simulink model "adc16_dbf_4fft"  (R2013a)
settings: Solver=ode45  StartTime=0.0  StopTime=2050  RelTol=1e-3
undefined symbols (not defined in the file): pfb_coeff_gen_calc
libraries: xbsIndex_r4 x1713, casper_library_misc x294, casper_library_delays x48, casper_library_pfbs x16, simulink x16, xps_library x1
(part 1 of 21)
settings Model: Creator=root  LastModifiedBy=root

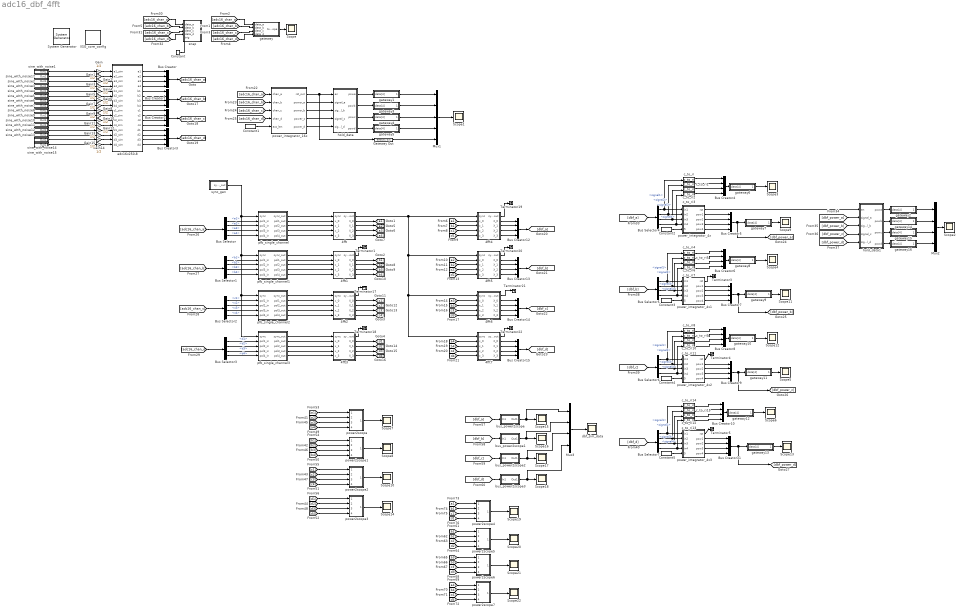
== system adc16_dbf_4fft ==
  " System Generator" : xbsIndex_r4/ System Generator  Tag=genX  xilinxfamily=Kintex7  part=xc7k325t  speed=-3  package=fbg676  synthesis_tool=XST  clock_wrapper=Clock Enables  directory=./netlist  proj_type=Project Navigator  Synth_file=XST Defaults  Impl_file=ISE Defaults  testbench=off  simulink_period=1  sysclk_period=10  dcm_input_clock_period=10  incr_netlist=off  trim_vbits=Everywhere in SubSystem  dbl_ovrd=According to Block Masks  core_generation=According to Block Masks  run_coregen=off  deprecated_control=off  eval_field=0  block_type=sysgen
  4fft : Subsystem
  4fft1 : Subsystem
  4fft2 : Subsystem
  4fft3 : Subsystem
  4fft4 : Subsystem
  4fft5 : Subsystem
  4fft6 : Subsystem
  4fft7 : Subsystem
  Bus Creator{,1..15} (16 alike) : BusCreator
  Bus Selector : BusSelector  OutputSignals=a1,a2,a3,a4
  Bus Selector1 : BusSelector  OutputSignals=b1,b2,b3,b4
  Bus Selector2 : BusSelector  OutputSignals=c1,c2,c3,c4
  Bus Selector3 : BusSelector  OutputSignals=d1,d2,d3,d4
  Bus Selector{4..7} (4 alike) : BusSelector  OutputSignals=signal1,signal2,signal3,signal4
  Constant : xbsIndex_r4/Constant  const=1  gui_display_data_type=Boolean  arith_type=Boolean  n_bits=16  bin_pt=14  preci_type=Single  exp_width=8  frac_width=24  explicit_period=off  period=1  equ=P=C  opselect=C  inp2=PCIN>>17  opr=+  inp1=P  carry=CIN  dbl_ovrd=off  block_type=constant
  Constant1 : xbsIndex_r4/Constant  const=255  gui_display_data_type=Fixed-point  arith_type=Unsigned  n_bits=10  bin_pt=0  preci_type=Single  exp_width=8  frac_width=24  explicit_period=off  period=1  equ=P=C  opselect=C  inp2=PCIN>>17  opr=+  inp1=P  carry=CIN  dbl_ovrd=off  block_type=constant
  Constant{2..5} (4 alike) : xbsIndex_r4/Constant  const=511  gui_display_data_type=Fixed-point  arith_type=Unsigned  n_bits=10  bin_pt=0  preci_type=Single  exp_width=8  frac_width=24  explicit_period=off  period=1  equ=P=C  opselect=C  inp2=PCIN>>17  opr=+  inp1=P  carry=CIN  dbl_ovrd=off  block_type=constant
  Gain{,1..15} (16 alike) : Gain  Gain=1/2
  Gateway Out : xbsIndex_r4/Gateway Out  inherit_from_input=off  hdl_port=on  timing_constraint=None  locs_specified=off  LOCs={}  UseAsDAC=off  DACChannel='1'  block_type=gatewayout
  Mux1 : Mux  Inputs=5
  Mux2 : Mux
  Mux3 : Mux
  Scope{,1..22} (23 alike) : Scope
      Scope10 settings: SaveName=ScopeData10
      Scope11 settings: SaveName=ScopeData4
      Scope12 settings: SaveName=ScopeData6
      Scope13 settings: SaveName=ScopeData7
      Scope14 settings: SaveName=ScopeData14
      Scope15 settings: SaveName=ScopeData15
      Scope16 settings: SaveName=ScopeData16
      Scope17 settings: SaveName=ScopeData17
      Scope18 settings: SaveName=ScopeData18
      Scope19 settings: SaveName=ScopeData19
      Scope2 settings: SaveName=ScopeData2
      Scope20 settings: SaveName=ScopeData20
      Scope21 settings: SaveName=ScopeData21
      Scope22 settings: SaveName=ScopeData22
      Scope3 settings: SaveName=ScopeData3
      Scope4 settings: SaveName=ScopeData11
      Scope5 settings: SaveName=ScopeData12
      Scope6 settings: SaveName=ScopeData13
      Scope7 settings: SaveName=ScopeData5
      Scope8 settings: SaveName=ScopeData8
      Scope9 settings: SaveName=ScopeData9
  Terminator{1,3..5,17..22} (10 alike) : Terminator
  XSG_core_config : xps_library/XSG_core_config  Tag=xps:xsg  hw_sys=ROACH2:sx475t  clk_src=adc0_clk  ROACH_clk_src=sys_clk  ROACH2_clk_src=adc0_clk  MKDIG_clk_src=sys_clk  clk_rate=240  sample_period=1  synthesis_tool=XST
  adc16x250-8 : Subsystem  Tag=xps:adc16  AncestorBlock=xps_library/ADCs/adc16x250-8  mask(ADC16){board_count=1, roach2_rev=2, zdok_rev=2}
      mask prompts: board_count "Number of ADC16 Boards"; roach2_rev "ROACH2 Revision"; zdok_rev "ZDOK Pinout Revision"
      mask help: 16-input ADC. When using one ADC16 board, it must be in ZDOK0.
      mask init:
      | % Only board_count is needed by init function
      | adc16_init(gcb, ...
      |     'board_count', board_count);
      settings: AttributesFormatString=r2 rev%<roach2_rev>\nzdok rev%<zdok_rev>
      mask Help:
      | This is the CASPER "yellow block" for the CASPER ADC16 board.  Each ADC
      | board has four ADC chips.  Each ADC chip accepts four inputs.  The four
      | 8-bit outputs from each ADC chip are concatenated into a 32-bit signal.
      mask TypeOptions board_count: 1 | 2
      mask TypeOptions roach2_rev: 1 | 2
      mask TypeOptions zdok_rev: 1 | 2
  bus_power2scope : Subsystem
  bus_power2scope1 : Subsystem
  bus_power2scope2 : Subsystem
  bus_power2scope3 : Subsystem
  c_to_ri{,1..15} (16 alike) : casper_library_misc/c_to_ri  n_bits=18  bin_pt=17
  dbf_sim_data : Scope
      settings: SaveName=dbf_sim_data
  gateway : Subsystem
  gateway1 : Subsystem
  gateway10 : Subsystem
  gateway11 : Subsystem
  gateway12 : Subsystem
  gateway13 : Subsystem
  gateway14 : Subsystem
  gateway15 : Subsystem
  gateway16 : Subsystem
  gateway2 : Subsystem
  gateway3 : Subsystem
  gateway4 : Subsystem
  gateway5 : Subsystem
  gateway6 : Subsystem
  gateway7 : Subsystem
  gateway8 : Subsystem
  gateway9 : Subsystem
  hold_data : Subsystem
  hold_data1 : Subsystem
  pfb_single_channel : Subsystem
  pfb_single_channel1 : Subsystem
  pfb_single_channel2 : Subsystem
  pfb_single_channel3 : Subsystem
  power2scope : Subsystem
  power2scope1 : Subsystem
  power2scope2 : Subsystem
  power2scope3 : Subsystem
  power2scope4 : Subsystem
  power2scope5 : Subsystem
  power2scope6 : Subsystem
  power2scope7 : Subsystem
  power_integrator_16x : Subsystem
  power_integrator_4x : Subsystem
  power_integrator_4x1 : Subsystem
  power_integrator_4x2 : Subsystem
  power_integrator_4x3 : Subsystem
  sine_with_noise1 : Subsystem
  sine_with_noise10 : Subsystem
  sine_with_noise11 : Subsystem
  sine_with_noise12 : Subsystem
  sine_with_noise13 : Subsystem
  sine_with_noise14 : Subsystem
  sine_with_noise15 : Subsystem
  sine_with_noise17 : Subsystem
  sine_with_noise2 : Subsystem
  sine_with_noise3 : Subsystem
  sine_with_noise4 : Subsystem
  sine_with_noise5 : Subsystem
  sine_with_noise6 : Subsystem
  sine_with_noise7 : Subsystem
  sine_with_noise8 : Subsystem
  sine_with_noise9 : Subsystem
  snap : Subsystem
  sync_gen : Subsystem  AncestorBlock=casper_library_misc/sync_gen  mask(sync_gen){sim_acc_len=4, fft_size=4, fft_simult_inputs=1, pfb_fir_taps=1, reorder_vec=[2 2 2], scale=32}
      mask prompts: sim_acc_len "Simulation Accumulation Length"; fft_size "FFT Size"; fft_simult_inputs "Simultaneous Inputs (FFT)"; pfb_fir_taps "Taps in pfb_fir (use 1 if no pfb_fir)"; reorder_vec "Reorder Orders (e.g. [2 2 2])"
      mask help:
      | This block computes the sync period based on system parameters as
      | described in Casper memo.  Detailed descritions of the block's
      | variables can be found in the 'Block Documentation' section of
      | the CASPER wiki.
      mask init:
      | sync_gen_init(gcb, ...
      |     'sim_acc_len', sim_acc_len, ...
      |     'fft_size', fft_size, ...
      |     'fft_simult_inputs', fft_simult_inputs,...
      |     'pfb_fir_taps', pfb_fir_taps, ...
      |     'reorder_vec', reorder_vec, ...
      |     'scale', scale);
      settings: AttributesFormatString=sim_sync_period=1024
      mask Help:
      | SyncPeriod=LCM(reorder_vec)*(acc_num)*(pfb_fir_len)*(fft_size/fft_simult_inputs)
      | 
      | See CASPER sync pulse memo for more details.
  wires:
  adc16x250-8/3(a3) -> Bus Creator/3
  adc16x250-8/2(a2) -> Bus Creator/2
  adc16x250-8/4(a4) -> Bus Creator/4
  Constant/1 -> snap/5(trig)
  gateway/1(to_scope) -> Scope/1
  sine_with_noise1/1(Out1) -> Gain/1
  Gain/1 -> adc16x250-8/1(a1_sim)
  Gain1/1 -> adc16x250-8/2(a2_sim)
  Gain2/1 -> adc16x250-8/3(a3_sim)
  Gain3/1 -> adc16x250-8/4(a4_sim)
  Gain4/1 -> adc16x250-8/5(b1_sim)
  Gain5/1 -> adc16x250-8/6(b2_sim)
  Gain6/1 -> adc16x250-8/7(b3_sim)
  Gain7/1 -> adc16x250-8/8(b4_sim)
  Gain10/1 -> adc16x250-8/11(c3_sim)
  Gain8/1 -> adc16x250-8/9(c1_sim)
  Gain12/1 -> adc16x250-8/13(d1_sim)
  Gain15/1 -> adc16x250-8/16(d4_sim)
  Gain11/1 -> adc16x250-8/12(c4_sim)
  Gain14/1 -> adc16x250-8/15(d3_sim)
  Gain9/1 -> adc16x250-8/10(c2_sim)
  Gain13/1 -> adc16x250-8/14(d2_sim)
  adc16x250-8/1(a1) -> Bus Creator/1
  Bus Creator/1 -> [adc16_chan_a]
  power_integrator_16x/2(power_a) -> hold_data/2(signal_a)
  hold_data/1(powa) -> gateway1/1(data[4])
  power_integrator_16x/1(rst_out) -> Gateway Out/1, hold_data/1(en)
  Mux1/1 -> Scope1/1
  Gateway Out/1 -> Mux1/5
  [adc16_chan_a] -> Bus Selector/1
  [adc16_chan_a] -> gateway/1(data_a)
  sync_gen/1(sync_out) -> pfb_single_channel3/1(sync), pfb_single_channel2/1(sync), pfb_single_channel1/1(sync), pfb_single_channel/1(sync)
  Bus Selector/4 -> pfb_single_channel/5(pol4_in)  "<a4>"
  Bus Selector/2 -> pfb_single_channel/3(pol2_in)  "<a2>"
  Bus Selector/1 -> pfb_single_channel/2(pol1_in)  "<a1>"
  Bus Selector/3 -> pfb_single_channel/4(pol3_in)  "<a3>"
  sine_with_noise17/1(Out1) -> Gain1/1
  sine_with_noise2/1(Out1) -> Gain2/1
  sine_with_noise3/1(Out1) -> Gain3/1
  sine_with_noise4/1(Out1) -> Gain4/1
  sine_with_noise5/1(Out1) -> Gain5/1
  sine_with_noise6/1(Out1) -> Gain6/1
  sine_with_noise7/1(Out1) -> Gain7/1
  sine_with_noise8/1(Out1) -> Gain8/1
  sine_with_noise9/1(Out1) -> Gain9/1
  sine_with_noise10/1(Out1) -> Gain10/1
  sine_with_noise11/1(Out1) -> Gain11/1
  sine_with_noise12/1(Out1) -> Gain12/1
  sine_with_noise13/1(Out1) -> Gain13/1
  sine_with_noise14/1(Out1) -> Gain14/1
  sine_with_noise15/1(Out1) -> Gain15/1
  pfb_single_channel/1(sync_out) -> 4fft/1(sync)
  4fft/1(sync_out) -> 4fft4/1(sync), 4fft5/1(sync), 4fft6/1(sync), 4fft7/1(sync)
  [adc16_chan_b] -> Bus Selector1/1
  pfb_single_channel1/2(pol1_out) -> 4fft1/2(x_0)
  pfb_single_channel1/4(pol3_out) -> 4fft1/4(x_2)
  pfb_single_channel1/3(pol2_out) -> 4fft1/3(x_1)
  pfb_single_channel1/5(pol4_out) -> 4fft1/5(x_3)
  Bus Selector1/4 -> pfb_single_channel1/5(pol4_in)  "<b4>"
  Bus Selector1/2 -> pfb_single_channel1/3(pol2_in)  "<b2>"
  Bus Selector1/1 -> pfb_single_channel1/2(pol1_in)  "<b1>"
  Bus Selector1/3 -> pfb_single_channel1/4(pol3_in)  "<b3>"
  pfb_single_channel1/1(sync_out) -> 4fft1/1(sync)
  4fft1/1(sync_out) -> Terminator1/1
  [adc16_chan_c] -> Bus Selector2/1
  pfb_single_channel2/2(pol1_out) -> 4fft2/2(x_0)
  pfb_single_channel2/4(pol3_out) -> 4fft2/4(x_2)
  pfb_single_channel2/3(pol2_out) -> 4fft2/3(x_1)
  pfb_single_channel2/5(pol4_out) -> 4fft2/5(x_3)
  Bus Selector2/4 -> pfb_single_channel2/5(pol4_in)  "<c4>"
  Bus Selector2/2 -> pfb_single_channel2/3(pol2_in)  "<c2>"
  Bus Selector2/1 -> pfb_single_channel2/2(pol1_in)  "<c1>"
  Bus Selector2/3 -> pfb_single_channel2/4(pol3_in)  "<c3>"
  pfb_single_channel2/1(sync_out) -> 4fft2/1(sync)
  4fft2/1(sync_out) -> Terminator17/1
  [adc16_chan_d] -> Bus Selector3/1
  pfb_single_channel3/2(pol1_out) -> 4fft3/2(x_0)
  pfb_single_channel3/4(pol3_out) -> 4fft3/4(x_2)
  pfb_single_channel3/3(pol2_out) -> 4fft3/3(x_1)
  pfb_single_channel3/5(pol4_out) -> 4fft3/5(x_3)
  Bus Selector3/4 -> pfb_single_channel3/5(pol4_in)  "<d4>"
  Bus Selector3/2 -> pfb_single_channel3/3(pol2_in)  "<d2>"
  Bus Selector3/1 -> pfb_single_channel3/2(pol1_in)  "<d1>"
  Bus Selector3/3 -> pfb_single_channel3/4(pol3_in)  "<d3>"
  pfb_single_channel3/1(sync_out) -> 4fft3/1(sync)
  4fft3/1(sync_out) -> Terminator18/1
  4fft/5(X_3) -> [a4]
  4fft/2(X_0) -> [a1]
  4fft/4(X_2) -> [a3]
  4fft/3(X_1) -> [a2]
  4fft2/3(X_1) -> [c2]
  4fft2/2(X_0) -> [c1]
  4fft2/4(X_2) -> [c3]
  4fft2/5(X_3) -> [c4]
  4fft3/2(X_0) -> [d1]
  4fft3/3(X_1) -> [d2]
  4fft3/4(X_2) -> [d3]
  4fft3/5(X_3) -> [d4]
  4fft1/2(X_0) -> [b1]
  4fft1/3(X_1) -> [b2]
  4fft1/4(X_2) -> [b3]
  4fft1/5(X_3) -> [b4]
  [a1] -> 4fft4/2(x_0)
  [b1] -> 4fft4/3(x_1)
  [c1] -> 4fft4/4(x_2)
  [d1] -> 4fft4/5(x_3)
  4fft4/1(sync_out) -> Terminator19/1
  [a2] -> 4fft5/2(x_0)
  [b2] -> 4fft5/3(x_1)
  [c2] -> 4fft5/4(x_2)
  [d2] -> 4fft5/5(x_3)
  [a3] -> 4fft6/2(x_0)
  [b3] -> 4fft6/3(x_1)
  [c3] -> 4fft6/4(x_2)
  [d3] -> 4fft6/5(x_3)
  [a4] -> 4fft7/2(x_0)
  [b4] -> 4fft7/3(x_1)
  [c4] -> 4fft7/4(x_2)
  [d4] -> 4fft7/5(x_3)
  4fft5/1(sync_out) -> Terminator20/1
  4fft6/1(sync_out) -> Terminator21/1
  4fft7/1(sync_out) -> Terminator22/1
  Constant1/1 -> power_integrator_16x/5(acc_len)
  adc16x250-8/8(b4) -> Bus Creator1/4
  adc16x250-8/6(b2) -> Bus Creator1/2
  adc16x250-8/7(b3) -> Bus Creator1/3
  adc16x250-8/5(b1) -> Bus Creator1/1
  adc16x250-8/12(c4) -> Bus Creator2/4
  adc16x250-8/11(c3) -> Bus Creator2/3
  adc16x250-8/10(c2) -> Bus Creator2/2
  adc16x250-8/9(c1) -> Bus Creator2/1
  adc16x250-8/15(d3) -> Bus Creator3/3
  adc16x250-8/16(d4) -> Bus Creator3/4
  adc16x250-8/14(d2) -> Bus Creator3/2
  adc16x250-8/13(d1) -> Bus Creator3/1
  Bus Creator1/1 -> [adc16_chan_b]
  Bus Creator2/1 -> [adc16_chan_c]
  Bus Creator3/1 -> [adc16_chan_d]
  [adc16_chan_a] -> power_integrator_16x/1(chan_a)
  [adc16_chan_b] -> power_integrator_16x/2(chan_b)
  [adc16_chan_c] -> power_integrator_16x/3(chan_c)
  [adc16_chan_d] -> power_integrator_16x/4(chan_d)
  power_integrator_16x/3(power_b) -> hold_data/3(signal_b)
  power_integrator_16x/4(power_c) -> hold_data/4(signal_c)
  power_integrator_16x/5(power_d) -> hold_data/5(signal_d)
  hold_data/2(powb) -> gateway3/1(data[4])
  hold_data/3(powc) -> gateway4/1(data[4])
  hold_data/4(powd) -> gateway5/1(data[4])
  gateway1/1(to_scope) -> Mux1/1
  gateway3/1(to_scope) -> Mux1/2
  gateway4/1(to_scope) -> Mux1/3
  gateway5/1(to_scope) -> Mux1/4
  [adc16_chan_b] -> gateway/2(data_b)
  [adc16_chan_c] -> gateway/3(data_c)
  [adc16_chan_d] -> gateway/4(data_d)
  [adc16_chan_c] -> snap/3(data_c)
  [adc16_chan_b] -> snap/2(data_b)
  [adc16_chan_d] -> snap/4(data_d)
  [adc16_chan_a] -> snap/1(data_a)
  pfb_single_channel/2(pol1_out) -> 4fft/2(x_0)
  pfb_single_channel/3(pol2_out) -> 4fft/3(x_1)
  pfb_single_channel/4(pol3_out) -> 4fft/4(x_2)
  pfb_single_channel/5(pol4_out) -> 4fft/5(x_3)
  Constant2/1 -> power_integrator_4x/5(acc_len)
  power_integrator_4x/1(rst) -> hold_data1/1(en)
  4fft4/3(X_1) -> Bus Creator12/2
  4fft4/4(X_2) -> Bus Creator12/3
  4fft4/2(X_0) -> Bus Creator12/1
  4fft4/5(X_3) -> Bus Creator12/4
  4fft5/5(X_3) -> Bus Creator13/4
  4fft5/4(X_2) -> Bus Creator13/3
  4fft5/2(X_0) -> Bus Creator13/1
  4fft5/3(X_1) -> Bus Creator13/2
  4fft6/2(X_0) -> Bus Creator14/1
  4fft6/3(X_1) -> Bus Creator14/2
  4fft6/4(X_2) -> Bus Creator14/3
  4fft6/5(X_3) -> Bus Creator14/4
  4fft7/5(X_3) -> Bus Creator15/4
  4fft7/2(X_0) -> Bus Creator15/1
  4fft7/3(X_1) -> Bus Creator15/2
  4fft7/4(X_2) -> Bus Creator15/3
  Bus Creator12/1 -> [dbf_a]
  Bus Creator13/1 -> [dbf_b]
  Bus Creator15/1 -> [dbf_d]
  [dbf_a] -> Bus Selector4/1
  [dbf_b] -> Bus Selector5/1
  [dbf_c] -> Bus Selector6/1
  [dbf_d] -> Bus Selector7/1
  Bus Selector4/1 -> c_to_ri/1, power_integrator_4x/1(in1)  "<signal1>"
  Bus Selector4/2 -> c_to_ri1/1, power_integrator_4x/2(in2)  "<signal2>"
  Bus Selector4/3 -> c_to_ri2/1, power_integrator_4x/3(in3)  "<signal3>"
  Bus Selector4/4 -> c_to_ri3/1, power_integrator_4x/4(in4)  "<signal4>"
  Constant3/1 -> power_integrator_4x1/5(acc_len)
  power_integrator_4x1/1(rst) -> Terminator3/1
  Bus Selector5/3 -> c_to_ri6/1, power_integrator_4x1/3(in3)  "<signal3>"
  Bus Selector5/2 -> c_to_ri5/1, power_integrator_4x1/2(in2)  "<signal2>"
  Bus Selector5/4 -> c_to_ri7/1, power_integrator_4x1/4(in4)  "<signal4>"
  Bus Selector5/1 -> power_integrator_4x1/1(in1), c_to_ri4/1  "<signal1>"
  Constant4/1 -> power_integrator_4x2/5(acc_len)
  power_integrator_4x2/1(rst) -> Terminator4/1
  Bus Selector6/3 -> c_to_ri10/1, power_integrator_4x2/3(in3)  "<signal3>"
  Bus Selector6/2 -> c_to_ri9/1, power_integrator_4x2/2(in2)  "<signal2>"
  Bus Selector6/4 -> c_to_ri11/1, power_integrator_4x2/4(in4)  "<signal4>"
  Bus Selector6/1 -> c_to_ri8/1, power_integrator_4x2/1(in1)  "<signal1>"
  Constant5/1 -> power_integrator_4x3/5(acc_len)
  power_integrator_4x3/1(rst) -> Terminator5/1
  Bus Selector7/3 -> c_to_ri12/1, power_integrator_4x3/3(in3)  "<signal3>"
  Bus Selector7/2 -> c_to_ri15/1, power_integrator_4x3/2(in2)  "<signal2>"
  Bus Selector7/4 -> c_to_ri13/1, power_integrator_4x3/4(in4)  "<signal4>"
  Bus Selector7/1 -> c_to_ri14/1, power_integrator_4x3/1(in1)  "<signal1>"
  power_integrator_4x/5(pow4) -> Bus Creator5/4
  power_integrator_4x/3(pow2) -> Bus Creator5/2
  power_integrator_4x/2(pow1) -> Bus Creator5/1
  power_integrator_4x/4(pow3) -> Bus Creator5/3
  Bus Creator4/1 -> gateway6/1(data[4])
  gateway6/1(to_scope) -> Scope3/1
  gateway7/1(to_scope) -> Scope9/1
  Bus Creator5/1 -> [dbf_power_a], gateway7/1(data[4])
  power_integrator_4x1/5(pow4) -> Bus Creator7/4
  power_integrator_4x1/3(pow2) -> Bus Creator7/2
  power_integrator_4x1/2(pow1) -> Bus Creator7/1
  power_integrator_4x1/4(pow3) -> Bus Creator7/3
  Bus Creator6/1 -> gateway8/1(data[4])
  gateway8/1(to_scope) -> Scope4/1
  gateway9/1(to_scope) -> Scope11/1
  Bus Creator7/1 -> [dbf_power_b], gateway9/1(data[4])
  power_integrator_4x2/5(pow4) -> Bus Creator9/4
  power_integrator_4x2/3(pow2) -> Bus Creator9/2
  power_integrator_4x2/2(pow1) -> Bus Creator9/1
  power_integrator_4x2/4(pow3) -> Bus Creator9/3
  Bus Creator8/1 -> gateway10/1(data[4])
  gateway10/1(to_scope) -> Scope12/1
  gateway11/1(to_scope) -> Scope5/1
  power_integrator_4x3/5(pow4) -> Bus Creator11/4
  power_integrator_4x3/3(pow2) -> Bus Creator11/2
  power_integrator_4x3/2(pow1) -> Bus Creator11/1
  power_integrator_4x3/4(pow3) -> Bus Creator11/3
  Bus Creator10/1 -> gateway12/1(data[4])
  gateway12/1(to_scope) -> Scope6/1
  gateway13/1(to_scope) -> Scope13/1
  Bus Creator14/1 -> [dbf_c]
  c_to_ri/1 -> Bus Creator4/1
  c_to_ri4/2 -> Bus Creator6/1
  c_to_ri5/2 -> Bus Creator6/2
  c_to_ri6/2 -> Bus Creator6/3
  c_to_ri7/2 -> Bus Creator6/4
  c_to_ri11/2 -> Bus Creator8/4
  c_to_ri10/2 -> Bus Creator8/3
  c_to_ri9/2 -> Bus Creator8/2
  c_to_ri8/2 -> Bus Creator8/1
  c_to_ri13/2 -> Bus Creator10/4
  c_to_ri12/2 -> Bus Creator10/3
  c_to_ri15/2 -> Bus Creator10/2
  c_to_ri14/2 -> Bus Creator10/1
  Bus Creator9/1 -> [dbf_power_c], gateway11/1(data[4])
  Bus Creator11/1 -> [dbf_power_d], gateway13/1(data[4])
  [dbf_power_a] -> hold_data1/2(signal_a)
  [dbf_power_b] -> hold_data1/3(signal_b)
  [dbf_power_c] -> hold_data1/4(signal_c)
  [dbf_power_d] -> hold_data1/5(signal_d)
  gateway2/1(to_scope) -> Mux2/1
  gateway14/1(to_scope) -> Mux2/2
  gateway15/1(to_scope) -> Mux2/3
  gateway16/1(to_scope) -> Mux2/4
  hold_data1/1(powa) -> gateway2/1(data[4])
  hold_data1/2(powb) -> gateway14/1(data[4])
  hold_data1/3(powc) -> gateway15/1(data[4])
  hold_data1/4(powd) -> gateway16/1(data[4])
  Mux2/1 -> Scope2/1
  c_to_ri1/1 -> Bus Creator4/2
  c_to_ri2/1 -> Bus Creator4/3
  c_to_ri3/1 -> Bus Creator4/4
  [dbf_a] -> bus_power2scope/1(In1)
  bus_power2scope/1(Out1) -> Mux3/1, Scope15/1
  [a1] -> power2scope/1(In1)
  [a2] -> power2scope/2(In2)
  [a3] -> power2scope/3(In3)
  [a4] -> power2scope/4(In4)
  power2scope/1(Out1) -> Scope7/1
  [dbf_b] -> bus_power2scope1/1(In1)
  [dbf_c] -> bus_power2scope2/1(In1)
  [dbf_d] -> bus_power2scope3/1(In1)
  bus_power2scope1/1(Out1) -> Mux3/2, Scope16/1
  bus_power2scope2/1(Out1) -> Mux3/3, Scope17/1
  bus_power2scope3/1(Out1) -> Mux3/4, Scope18/1
  power2scope1/1(Out1) -> Scope8/1
  [b3] -> power2scope1/3(In3)
  [b2] -> power2scope1/2(In2)
  [b1] -> power2scope1/1(In1)
  [b4] -> power2scope1/4(In4)
  [c1] -> power2scope2/1(In1)
  [c2] -> power2scope2/2(In2)
  [c3] -> power2scope2/3(In3)
  [c4] -> power2scope2/4(In4)
  [d2] -> power2scope3/2(In2)
  [d1] -> power2scope3/1(In1)
  [d3] -> power2scope3/3(In3)
  [d4] -> power2scope3/4(In4)
  power2scope3/1(Out1) -> Scope14/1
  power2scope2/1(Out1) -> Scope10/1
  [a1] -> power2scope4/1(In1)
  [b1] -> power2scope4/2(In2)
  [c1] -> power2scope4/3(In3)
  [d1] -> power2scope4/4(In4)
  [a2] -> power2scope5/1(In1)
  [b2] -> power2scope5/2(In2)
  [c2] -> power2scope5/3(In3)
  [d2] -> power2scope5/4(In4)
  [a3] -> power2scope6/1(In1)
  [b3] -> power2scope6/2(In2)
  [c3] -> power2scope6/3(In3)
  [d3] -> power2scope6/4(In4)
  [a4] -> power2scope7/1(In1)
  [b4] -> power2scope7/2(In2)
  [c4] -> power2scope7/3(In3)
  [d4] -> power2scope7/4(In4)
  power2scope4/1(Out1) -> Scope19/1
  power2scope5/1(Out1) -> Scope20/1
  power2scope6/1(Out1) -> Scope21/1
  power2scope7/1(Out1) -> Scope22/1
  Mux3/1 -> dbf_sim_data/1

== system adc16_dbf_4fft/4fft ==
  sync : Inport
  x_0 : Inport  Port=2
  x_1 : Inport  Port=3
  x_2 : Inport  Port=4
  x_3 : Inport  Port=5
  complex_addsub{,1..7} (8 alike) : casper_library_misc/complex_addsub  BitWidth=18  add_latency=2
  mult_j : Subsystem
  mult_jjj : Subsystem
  pipeline : Subsystem  AncestorBlock=casper_library_delays/pipeline  mask(pipeline){latency=4}
      mask help:
      | An explicitly laid-out delay line to avoid mapping to SRL16s
      | for use in pipelining to help achieve timing closure.
      mask init:
      | pipeline_init(gcb,'latency',latency);
      settings: AttributesFormatString=Latency = %<latency>
      mask Display:
      | port_label('input', 1, 'd');
      | port_label('output', 1, 'q');
      | disp(['Z^-', num2str(latency)]);
  pipeline1 : Subsystem  AncestorBlock=casper_library_delays/pipeline  mask(pipeline){latency=4}
      mask help:
      | An explicitly laid-out delay line to avoid mapping to SRL16s
      | for use in pipelining to help achieve timing closure.
      mask init:
      | pipeline_init(gcb,'latency',latency);
      settings: AttributesFormatString=Latency = %<latency>
      mask Display:
      | port_label('input', 1, 'd');
      | port_label('output', 1, 'q');
      | disp(['Z^-', num2str(latency)]);
  real2complex : Subsystem
  real2complex1 : Subsystem
  real2complex2 : Subsystem
  real2complex3 : Subsystem
  sync_out : Outport
  X_0 : Outport  Port=2
  X_1 : Outport  Port=3
  X_2 : Outport  Port=4
  X_3 : Outport  Port=5
  wires:
  x_0/1 -> real2complex/1(r)
  x_1/1 -> real2complex1/1(r)
  complex_addsub1/1 -> complex_addsub5/2, complex_addsub4/2
  complex_addsub/1 -> complex_addsub5/1, complex_addsub4/1
  complex_addsub2/2 -> complex_addsub7/1, complex_addsub6/1
  complex_addsub4/1 -> X_0/1
  complex_addsub5/2 -> X_2/1
  complex_addsub6/1 -> X_1/1
  complex_addsub7/1 -> X_3/1
  complex_addsub3/2 -> mult_jjj/1(a+jb), mult_j/1(a+jb)
  mult_j/1(ja-b) -> complex_addsub7/2
  mult_jjj/1(b-ja) -> complex_addsub6/2
  x_3/1 -> real2complex3/1(r)
  x_2/1 -> real2complex2/1(r)
  real2complex/1(c) -> complex_addsub2/1, complex_addsub/1
  real2complex1/1(c) -> complex_addsub3/1, complex_addsub1/1
  real2complex2/1(c) -> complex_addsub2/2, complex_addsub/2
  real2complex3/1(c) -> complex_addsub3/2, complex_addsub1/2
  sync/1 -> pipeline/1(d)
  pipeline/1(q) -> pipeline1/1(d)
  pipeline1/1(q) -> sync_out/1

== system adc16_dbf_4fft/4fft1 ==
  sync : Inport
  x_0 : Inport  Port=2
  x_1 : Inport  Port=3
  x_2 : Inport  Port=4
  x_3 : Inport  Port=5
  complex_addsub{,1..7} (8 alike) : casper_library_misc/complex_addsub  BitWidth=18  add_latency=2
  mult_j : Subsystem
  mult_jjj : Subsystem
  pipeline : Subsystem  AncestorBlock=casper_library_delays/pipeline  mask(pipeline){latency=4}
      mask help:
      | An explicitly laid-out delay line to avoid mapping to SRL16s
      | for use in pipelining to help achieve timing closure.
      mask init:
      | pipeline_init(gcb,'latency',latency);
      settings: AttributesFormatString=Latency = %<latency>
      mask Display:
      | port_label('input', 1, 'd');
      | port_label('output', 1, 'q');
      | disp(['Z^-', num2str(latency)]);
  pipeline1 : Subsystem  AncestorBlock=casper_library_delays/pipeline  mask(pipeline){latency=4}
      mask help:
      | An explicitly laid-out delay line to avoid mapping to SRL16s
      | for use in pipelining to help achieve timing closure.
      mask init:
      | pipeline_init(gcb,'latency',latency);
      settings: AttributesFormatString=Latency = %<latency>
      mask Display:
      | port_label('input', 1, 'd');
      | port_label('output', 1, 'q');
      | disp(['Z^-', num2str(latency)]);
  real2complex : Subsystem
  real2complex1 : Subsystem
  real2complex2 : Subsystem
  real2complex3 : Subsystem
  sync_out : Outport
  X_0 : Outport  Port=2
  X_1 : Outport  Port=3
  X_2 : Outport  Port=4
  X_3 : Outport  Port=5
  wires:
  pipeline1/1(q) -> sync_out/1
  pipeline/1(q) -> pipeline1/1(d)
  sync/1 -> pipeline/1(d)
  real2complex3/1(c) -> complex_addsub1/2, complex_addsub3/2
  real2complex2/1(c) -> complex_addsub/2, complex_addsub2/2
  real2complex1/1(c) -> complex_addsub1/1, complex_addsub3/1
  real2complex/1(c) -> complex_addsub/1, complex_addsub2/1
  x_2/1 -> real2complex2/1(r)
  x_3/1 -> real2complex3/1(r)
  mult_jjj/1(b-ja) -> complex_addsub6/2
  mult_j/1(ja-b) -> complex_addsub7/2
  complex_addsub3/2 -> mult_j/1(a+jb), mult_jjj/1(a+jb)
  complex_addsub7/1 -> X_3/1
  complex_addsub6/1 -> X_1/1
  complex_addsub5/2 -> X_2/1
  complex_addsub4/1 -> X_0/1
  complex_addsub2/2 -> complex_addsub6/1, complex_addsub7/1
  complex_addsub/1 -> complex_addsub4/1, complex_addsub5/1
  complex_addsub1/1 -> complex_addsub4/2, complex_addsub5/2
  x_1/1 -> real2complex1/1(r)
  x_0/1 -> real2complex/1(r)

== system adc16_dbf_4fft/4fft2 ==
  sync : Inport
  x_0 : Inport  Port=2
  x_1 : Inport  Port=3
  x_2 : Inport  Port=4
  x_3 : Inport  Port=5
  complex_addsub{,1..7} (8 alike) : casper_library_misc/complex_addsub  BitWidth=18  add_latency=2
  mult_j : Subsystem
  mult_jjj : Subsystem
  pipeline : Subsystem  AncestorBlock=casper_library_delays/pipeline  mask(pipeline){latency=4}
      mask help:
      | An explicitly laid-out delay line to avoid mapping to SRL16s
      | for use in pipelining to help achieve timing closure.
      mask init:
      | pipeline_init(gcb,'latency',latency);
      settings: AttributesFormatString=Latency = %<latency>
      mask Display:
      | port_label('input', 1, 'd');
      | port_label('output', 1, 'q');
      | disp(['Z^-', num2str(latency)]);
  pipeline1 : Subsystem  AncestorBlock=casper_library_delays/pipeline  mask(pipeline){latency=4}
      mask help:
      | An explicitly laid-out delay line to avoid mapping to SRL16s
      | for use in pipelining to help achieve timing closure.
      mask init:
      | pipeline_init(gcb,'latency',latency);
      settings: AttributesFormatString=Latency = %<latency>
      mask Display:
      | port_label('input', 1, 'd');
      | port_label('output', 1, 'q');
      | disp(['Z^-', num2str(latency)]);
  real2complex : Subsystem
  real2complex1 : Subsystem
  real2complex2 : Subsystem
  real2complex3 : Subsystem
  sync_out : Outport
  X_0 : Outport  Port=2
  X_1 : Outport  Port=3
  X_2 : Outport  Port=4
  X_3 : Outport  Port=5
  wires:
  x_0/1 -> real2complex/1(r)
  x_1/1 -> real2complex1/1(r)
  complex_addsub1/1 -> complex_addsub5/2, complex_addsub4/2
  complex_addsub/1 -> complex_addsub5/1, complex_addsub4/1
  complex_addsub2/2 -> complex_addsub7/1, complex_addsub6/1
  complex_addsub4/1 -> X_0/1
  complex_addsub5/2 -> X_2/1
  complex_addsub6/1 -> X_1/1
  complex_addsub7/1 -> X_3/1
  complex_addsub3/2 -> mult_jjj/1(a+jb), mult_j/1(a+jb)
  mult_j/1(ja-b) -> complex_addsub7/2
  mult_jjj/1(b-ja) -> complex_addsub6/2
  x_3/1 -> real2complex3/1(r)
  x_2/1 -> real2complex2/1(r)
  real2complex/1(c) -> complex_addsub2/1, complex_addsub/1
  real2complex1/1(c) -> complex_addsub3/1, complex_addsub1/1
  real2complex2/1(c) -> complex_addsub2/2, complex_addsub/2
  real2complex3/1(c) -> complex_addsub3/2, complex_addsub1/2
  sync/1 -> pipeline/1(d)
  pipeline/1(q) -> pipeline1/1(d)
  pipeline1/1(q) -> sync_out/1

== system adc16_dbf_4fft/4fft3 ==
  sync : Inport
  x_0 : Inport  Port=2
  x_1 : Inport  Port=3
  x_2 : Inport  Port=4
  x_3 : Inport  Port=5
  complex_addsub{,1..7} (8 alike) : casper_library_misc/complex_addsub  BitWidth=18  add_latency=2
  mult_j : Subsystem
  mult_jjj : Subsystem
  pipeline : Subsystem  AncestorBlock=casper_library_delays/pipeline  mask(pipeline){latency=4}
      mask help:
      | An explicitly laid-out delay line to avoid mapping to SRL16s
      | for use in pipelining to help achieve timing closure.
      mask init:
      | pipeline_init(gcb,'latency',latency);
      settings: AttributesFormatString=Latency = %<latency>
      mask Display:
      | port_label('input', 1, 'd');
      | port_label('output', 1, 'q');
      | disp(['Z^-', num2str(latency)]);
  pipeline1 : Subsystem  AncestorBlock=casper_library_delays/pipeline  mask(pipeline){latency=4}
      mask help:
      | An explicitly laid-out delay line to avoid mapping to SRL16s
      | for use in pipelining to help achieve timing closure.
      mask init:
      | pipeline_init(gcb,'latency',latency);
      settings: AttributesFormatString=Latency = %<latency>
      mask Display:
      | port_label('input', 1, 'd');
      | port_label('output', 1, 'q');
      | disp(['Z^-', num2str(latency)]);
  real2complex : Subsystem
  real2complex1 : Subsystem
  real2complex2 : Subsystem
  real2complex3 : Subsystem
  sync_out : Outport
  X_0 : Outport  Port=2
  X_1 : Outport  Port=3
  X_2 : Outport  Port=4
  X_3 : Outport  Port=5
  wires:
  pipeline1/1(q) -> sync_out/1
  pipeline/1(q) -> pipeline1/1(d)
  sync/1 -> pipeline/1(d)
  real2complex3/1(c) -> complex_addsub1/2, complex_addsub3/2
  real2complex2/1(c) -> complex_addsub/2, complex_addsub2/2
  real2complex1/1(c) -> complex_addsub1/1, complex_addsub3/1
  real2complex/1(c) -> complex_addsub/1, complex_addsub2/1
  x_2/1 -> real2complex2/1(r)
  x_3/1 -> real2complex3/1(r)
  mult_jjj/1(b-ja) -> complex_addsub6/2
  mult_j/1(ja-b) -> complex_addsub7/2
  complex_addsub3/2 -> mult_j/1(a+jb), mult_jjj/1(a+jb)
  complex_addsub7/1 -> X_3/1
  complex_addsub6/1 -> X_1/1
  complex_addsub5/2 -> X_2/1
  complex_addsub4/1 -> X_0/1
  complex_addsub2/2 -> complex_addsub6/1, complex_addsub7/1
  complex_addsub/1 -> complex_addsub4/1, complex_addsub5/1
  complex_addsub1/1 -> complex_addsub4/2, complex_addsub5/2
  x_1/1 -> real2complex1/1(r)
  x_0/1 -> real2complex/1(r)

== system adc16_dbf_4fft/4fft4 ==
  sync : Inport
  x_0 : Inport  Port=2
  x_1 : Inport  Port=3
  x_2 : Inport  Port=4
  x_3 : Inport  Port=5
  complex_addsub{,1..7} (8 alike) : casper_library_misc/complex_addsub  BitWidth=18  add_latency=2
  mult_j : Subsystem
  mult_jjj : Subsystem
  pipeline : Subsystem  AncestorBlock=casper_library_delays/pipeline  mask(pipeline){latency=4}
      mask help:
      | An explicitly laid-out delay line to avoid mapping to SRL16s
      | for use in pipelining to help achieve timing closure.
      mask init:
      | pipeline_init(gcb,'latency',latency);
      settings: AttributesFormatString=Latency = %<latency>
      mask Display:
      | port_label('input', 1, 'd');
      | port_label('output', 1, 'q');
      | disp(['Z^-', num2str(latency)]);
  pipeline1 : Subsystem  AncestorBlock=casper_library_delays/pipeline  mask(pipeline){latency=4}
      mask help:
      | An explicitly laid-out delay line to avoid mapping to SRL16s
      | for use in pipelining to help achieve timing closure.
      mask init:
      | pipeline_init(gcb,'latency',latency);
      settings: AttributesFormatString=Latency = %<latency>
      mask Display:
      | port_label('input', 1, 'd');
      | port_label('output', 1, 'q');
      | disp(['Z^-', num2str(latency)]);
  real2complex : Subsystem
  real2complex1 : Subsystem
  real2complex2 : Subsystem
  real2complex3 : Subsystem
  sync_out : Outport
  X_0 : Outport  Port=2
  X_1 : Outport  Port=3
  X_2 : Outport  Port=4
  X_3 : Outport  Port=5
  wires:
  x_0/1 -> real2complex/1(r)
  x_1/1 -> real2complex1/1(r)
  complex_addsub1/1 -> complex_addsub5/2, complex_addsub4/2
  complex_addsub/1 -> complex_addsub5/1, complex_addsub4/1
  complex_addsub2/2 -> complex_addsub7/1, complex_addsub6/1
  complex_addsub4/1 -> X_0/1
  complex_addsub5/2 -> X_2/1
  complex_addsub6/1 -> X_1/1
  complex_addsub7/1 -> X_3/1
  complex_addsub3/2 -> mult_jjj/1(a+jb), mult_j/1(a+jb)
  mult_j/1(ja-b) -> complex_addsub7/2
  mult_jjj/1(b-ja) -> complex_addsub6/2
  x_3/1 -> real2complex3/1(r)
  x_2/1 -> real2complex2/1(r)
  real2complex/1(c) -> complex_addsub2/1, complex_addsub/1
  real2complex1/1(c) -> complex_addsub3/1, complex_addsub1/1
  real2complex2/1(c) -> complex_addsub2/2, complex_addsub/2
  real2complex3/1(c) -> complex_addsub3/2, complex_addsub1/2
  sync/1 -> pipeline/1(d)
  pipeline/1(q) -> pipeline1/1(d)
  pipeline1/1(q) -> sync_out/1

== system adc16_dbf_4fft/4fft5 ==
  sync : Inport
  x_0 : Inport  Port=2
  x_1 : Inport  Port=3
  x_2 : Inport  Port=4
  x_3 : Inport  Port=5
  complex_addsub{,1..7} (8 alike) : casper_library_misc/complex_addsub  BitWidth=18  add_latency=2
  mult_j : Subsystem
  mult_jjj : Subsystem
  pipeline : Subsystem  AncestorBlock=casper_library_delays/pipeline  mask(pipeline){latency=4}
      mask help:
      | An explicitly laid-out delay line to avoid mapping to SRL16s
      | for use in pipelining to help achieve timing closure.
      mask init:
      | pipeline_init(gcb,'latency',latency);
      settings: AttributesFormatString=Latency = %<latency>
      mask Display:
      | port_label('input', 1, 'd');
      | port_label('output', 1, 'q');
      | disp(['Z^-', num2str(latency)]);
  pipeline1 : Subsystem  AncestorBlock=casper_library_delays/pipeline  mask(pipeline){latency=4}
      mask help:
      | An explicitly laid-out delay line to avoid mapping to SRL16s
      | for use in pipelining to help achieve timing closure.
      mask init:
      | pipeline_init(gcb,'latency',latency);
      settings: AttributesFormatString=Latency = %<latency>
      mask Display:
      | port_label('input', 1, 'd');
      | port_label('output', 1, 'q');
      | disp(['Z^-', num2str(latency)]);
  real2complex : Subsystem
  real2complex1 : Subsystem
  real2complex2 : Subsystem
  real2complex3 : Subsystem
  sync_out : Outport
  X_0 : Outport  Port=2
  X_1 : Outport  Port=3
  X_2 : Outport  Port=4
  X_3 : Outport  Port=5
  wires:
  pipeline1/1(q) -> sync_out/1
  pipeline/1(q) -> pipeline1/1(d)
  sync/1 -> pipeline/1(d)
  real2complex3/1(c) -> complex_addsub1/2, complex_addsub3/2
  real2complex2/1(c) -> complex_addsub/2, complex_addsub2/2
  real2complex1/1(c) -> complex_addsub1/1, complex_addsub3/1
  real2complex/1(c) -> complex_addsub/1, complex_addsub2/1
  x_2/1 -> real2complex2/1(r)
  x_3/1 -> real2complex3/1(r)
  mult_jjj/1(b-ja) -> complex_addsub6/2
  mult_j/1(ja-b) -> complex_addsub7/2
  complex_addsub3/2 -> mult_j/1(a+jb), mult_jjj/1(a+jb)
  complex_addsub7/1 -> X_3/1
  complex_addsub6/1 -> X_1/1
  complex_addsub5/2 -> X_2/1
  complex_addsub4/1 -> X_0/1
  complex_addsub2/2 -> complex_addsub6/1, complex_addsub7/1
  complex_addsub/1 -> complex_addsub4/1, complex_addsub5/1
  complex_addsub1/1 -> complex_addsub4/2, complex_addsub5/2
  x_1/1 -> real2complex1/1(r)
  x_0/1 -> real2complex/1(r)

== system adc16_dbf_4fft/4fft6 ==
  sync : Inport
  x_0 : Inport  Port=2
  x_1 : Inport  Port=3
  x_2 : Inport  Port=4
  x_3 : Inport  Port=5
  complex_addsub{,1..7} (8 alike) : casper_library_misc/complex_addsub  BitWidth=18  add_latency=2
  mult_j : Subsystem
  mult_jjj : Subsystem
  pipeline : Subsystem  AncestorBlock=casper_library_delays/pipeline  mask(pipeline){latency=4}
      mask help:
      | An explicitly laid-out delay line to avoid mapping to SRL16s
      | for use in pipelining to help achieve timing closure.
      mask init:
      | pipeline_init(gcb,'latency',latency);
      settings: AttributesFormatString=Latency = %<latency>
      mask Display:
      | port_label('input', 1, 'd');
      | port_label('output', 1, 'q');
      | disp(['Z^-', num2str(latency)]);
  pipeline1 : Subsystem  AncestorBlock=casper_library_delays/pipeline  mask(pipeline){latency=4}
      mask help:
      | An explicitly laid-out delay line to avoid mapping to SRL16s
      | for use in pipelining to help achieve timing closure.
      mask init:
      | pipeline_init(gcb,'latency',latency);
      settings: AttributesFormatString=Latency = %<latency>
      mask Display:
      | port_label('input', 1, 'd');
      | port_label('output', 1, 'q');
      | disp(['Z^-', num2str(latency)]);
  real2complex : Subsystem
  real2complex1 : Subsystem
  real2complex2 : Subsystem
  real2complex3 : Subsystem
  sync_out : Outport
  X_0 : Outport  Port=2
  X_1 : Outport  Port=3
  X_2 : Outport  Port=4
  X_3 : Outport  Port=5
  wires:
  x_0/1 -> real2complex/1(r)
  x_1/1 -> real2complex1/1(r)
  complex_addsub1/1 -> complex_addsub5/2, complex_addsub4/2
  complex_addsub/1 -> complex_addsub5/1, complex_addsub4/1
  complex_addsub2/2 -> complex_addsub7/1, complex_addsub6/1
  complex_addsub4/1 -> X_0/1
  complex_addsub5/2 -> X_2/1
  complex_addsub6/1 -> X_1/1
  complex_addsub7/1 -> X_3/1
  complex_addsub3/2 -> mult_jjj/1(a+jb), mult_j/1(a+jb)
  mult_j/1(ja-b) -> complex_addsub7/2
  mult_jjj/1(b-ja) -> complex_addsub6/2
  x_3/1 -> real2complex3/1(r)
  x_2/1 -> real2complex2/1(r)
  real2complex/1(c) -> complex_addsub2/1, complex_addsub/1
  real2complex1/1(c) -> complex_addsub3/1, complex_addsub1/1
  real2complex2/1(c) -> complex_addsub2/2, complex_addsub/2
  real2complex3/1(c) -> complex_addsub3/2, complex_addsub1/2
  sync/1 -> pipeline/1(d)
  pipeline/1(q) -> pipeline1/1(d)
  pipeline1/1(q) -> sync_out/1

== system adc16_dbf_4fft/4fft7 ==
  sync : Inport
  x_0 : Inport  Port=2
  x_1 : Inport  Port=3
  x_2 : Inport  Port=4
  x_3 : Inport  Port=5
  complex_addsub{,1..7} (8 alike) : casper_library_misc/complex_addsub  BitWidth=18  add_latency=2
  mult_j : Subsystem
  mult_jjj : Subsystem
  pipeline : Subsystem  AncestorBlock=casper_library_delays/pipeline  mask(pipeline){latency=4}
      mask help:
      | An explicitly laid-out delay line to avoid mapping to SRL16s
      | for use in pipelining to help achieve timing closure.
      mask init:
      | pipeline_init(gcb,'latency',latency);
      settings: AttributesFormatString=Latency = %<latency>
      mask Display:
      | port_label('input', 1, 'd');
      | port_label('output', 1, 'q');
      | disp(['Z^-', num2str(latency)]);
  pipeline1 : Subsystem  AncestorBlock=casper_library_delays/pipeline  mask(pipeline){latency=4}
      mask help:
      | An explicitly laid-out delay line to avoid mapping to SRL16s
      | for use in pipelining to help achieve timing closure.
      mask init:
      | pipeline_init(gcb,'latency',latency);
      settings: AttributesFormatString=Latency = %<latency>
      mask Display:
      | port_label('input', 1, 'd');
      | port_label('output', 1, 'q');
      | disp(['Z^-', num2str(latency)]);
  real2complex : Subsystem
  real2complex1 : Subsystem
  real2complex2 : Subsystem
  real2complex3 : Subsystem
  sync_out : Outport
  X_0 : Outport  Port=2
  X_1 : Outport  Port=3
  X_2 : Outport  Port=4
  X_3 : Outport  Port=5
  wires:
  pipeline1/1(q) -> sync_out/1
  pipeline/1(q) -> pipeline1/1(d)
  sync/1 -> pipeline/1(d)
  real2complex3/1(c) -> complex_addsub1/2, complex_addsub3/2
  real2complex2/1(c) -> complex_addsub/2, complex_addsub2/2
  real2complex1/1(c) -> complex_addsub1/1, complex_addsub3/1
  real2complex/1(c) -> complex_addsub/1, complex_addsub2/1
  x_2/1 -> real2complex2/1(r)
  x_3/1 -> real2complex3/1(r)
  mult_jjj/1(b-ja) -> complex_addsub6/2
  mult_j/1(ja-b) -> complex_addsub7/2
  complex_addsub3/2 -> mult_j/1(a+jb), mult_jjj/1(a+jb)
  complex_addsub7/1 -> X_3/1
  complex_addsub6/1 -> X_1/1
  complex_addsub5/2 -> X_2/1
  complex_addsub4/1 -> X_0/1
  complex_addsub2/2 -> complex_addsub6/1, complex_addsub7/1
  complex_addsub/1 -> complex_addsub4/1, complex_addsub5/1
  complex_addsub1/1 -> complex_addsub4/2, complex_addsub5/2
  x_1/1 -> real2complex1/1(r)
  x_0/1 -> real2complex/1(r)

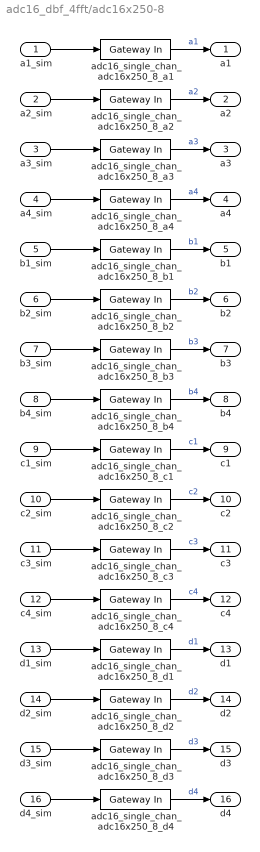
== system adc16_dbf_4fft/adc16x250-8 ==
  a1_sim : Inport
  a2_sim : Inport  Port=2
  a3_sim : Inport  Port=3
  a4_sim : Inport  Port=4
  b1_sim : Inport  Port=5
  b2_sim : Inport  Port=6
  b3_sim : Inport  Port=7
  b4_sim : Inport  Port=8
  c1_sim : Inport  Port=9
  c2_sim : Inport  Port=10
  c3_sim : Inport  Port=11
  c4_sim : Inport  Port=12
  d1_sim : Inport  Port=13
  d2_sim : Inport  Port=14
  d3_sim : Inport  Port=15
  d4_sim : Inport  Port=16
  adc16_single_chan_adc16x250_8_a{1..4} (4 alike) : xbsIndex_r4/Gateway In  gui_display_data_type=Fixed-point  arith_type="Signed  (2's comp)"  n_bits=8  bin_pt=7  preci_type=Single  exp_width=8  frac_width=24  quantization="Round  (unbiased: +/- Inf)"  overflow=Saturate  period=1  dbl_ovrd=off  timing_constraint=None  locs_specified=off  LOCs={}  UseAsADC=off  ADCChannel='1'  inherit_from_input=off  hdl_port=on  block_type=gatewayin
  adc16_single_chan_adc16x250_8_b{1..4} (4 alike) : xbsIndex_r4/Gateway In  gui_display_data_type=Fixed-point  arith_type="Signed  (2's comp)"  n_bits=8  bin_pt=7  preci_type=Single  exp_width=8  frac_width=24  quantization="Round  (unbiased: +/- Inf)"  overflow=Saturate  period=1  dbl_ovrd=off  timing_constraint=None  locs_specified=off  LOCs={}  UseAsADC=off  ADCChannel='1'  inherit_from_input=off  hdl_port=on  block_type=gatewayin
  adc16_single_chan_adc16x250_8_c{1..4} (4 alike) : xbsIndex_r4/Gateway In  gui_display_data_type=Fixed-point  arith_type="Signed  (2's comp)"  n_bits=8  bin_pt=7  preci_type=Single  exp_width=8  frac_width=24  quantization="Round  (unbiased: +/- Inf)"  overflow=Saturate  period=1  dbl_ovrd=off  timing_constraint=None  locs_specified=off  LOCs={}  UseAsADC=off  ADCChannel='1'  inherit_from_input=off  hdl_port=on  block_type=gatewayin
  adc16_single_chan_adc16x250_8_d{1..4} (4 alike) : xbsIndex_r4/Gateway In  gui_display_data_type=Fixed-point  arith_type="Signed  (2's comp)"  n_bits=8  bin_pt=7  preci_type=Single  exp_width=8  frac_width=24  quantization="Round  (unbiased: +/- Inf)"  overflow=Saturate  period=1  dbl_ovrd=off  timing_constraint=None  locs_specified=off  LOCs={}  UseAsADC=off  ADCChannel='1'  inherit_from_input=off  hdl_port=on  block_type=gatewayin
  a1 : Outport
  a2 : Outport  Port=2
  a3 : Outport  Port=3
  a4 : Outport  Port=4
  b1 : Outport  Port=5
  b2 : Outport  Port=6
  b3 : Outport  Port=7
  b4 : Outport  Port=8
  c1 : Outport  Port=9
  c2 : Outport  Port=10
  c3 : Outport  Port=11
  c4 : Outport  Port=12
  d1 : Outport  Port=13
  d2 : Outport  Port=14
  d3 : Outport  Port=15
  d4 : Outport  Port=16
  wires:
  a1_sim/1 -> adc16_single_chan_adc16x250_8_a1/1
  adc16_single_chan_adc16x250_8_a1/1 -> a1/1  "a1"
  a2_sim/1 -> adc16_single_chan_adc16x250_8_a2/1
  adc16_single_chan_adc16x250_8_a2/1 -> a2/1  "a2"
  a3_sim/1 -> adc16_single_chan_adc16x250_8_a3/1
  adc16_single_chan_adc16x250_8_a3/1 -> a3/1  "a3"
  a4_sim/1 -> adc16_single_chan_adc16x250_8_a4/1
  adc16_single_chan_adc16x250_8_a4/1 -> a4/1  "a4"
  b1_sim/1 -> adc16_single_chan_adc16x250_8_b1/1
  adc16_single_chan_adc16x250_8_b1/1 -> b1/1  "b1"
  b2_sim/1 -> adc16_single_chan_adc16x250_8_b2/1
  adc16_single_chan_adc16x250_8_b2/1 -> b2/1  "b2"
  b3_sim/1 -> adc16_single_chan_adc16x250_8_b3/1
  adc16_single_chan_adc16x250_8_b3/1 -> b3/1  "b3"
  b4_sim/1 -> adc16_single_chan_adc16x250_8_b4/1
  adc16_single_chan_adc16x250_8_b4/1 -> b4/1  "b4"
  c1_sim/1 -> adc16_single_chan_adc16x250_8_c1/1
  adc16_single_chan_adc16x250_8_c1/1 -> c1/1  "c1"
  c2_sim/1 -> adc16_single_chan_adc16x250_8_c2/1
  adc16_single_chan_adc16x250_8_c2/1 -> c2/1  "c2"
  c3_sim/1 -> adc16_single_chan_adc16x250_8_c3/1
  adc16_single_chan_adc16x250_8_c3/1 -> c3/1  "c3"
  c4_sim/1 -> adc16_single_chan_adc16x250_8_c4/1
  adc16_single_chan_adc16x250_8_c4/1 -> c4/1  "c4"
  d1_sim/1 -> adc16_single_chan_adc16x250_8_d1/1
  adc16_single_chan_adc16x250_8_d1/1 -> d1/1  "d1"
  d2_sim/1 -> adc16_single_chan_adc16x250_8_d2/1
  adc16_single_chan_adc16x250_8_d2/1 -> d2/1  "d2"
  d3_sim/1 -> adc16_single_chan_adc16x250_8_d3/1
  adc16_single_chan_adc16x250_8_d3/1 -> d3/1  "d3"
  d4_sim/1 -> adc16_single_chan_adc16x250_8_d4/1
  adc16_single_chan_adc16x250_8_d4/1 -> d4/1  "d4"

== system adc16_dbf_4fft/bus_power2scope ==
  In1 : Inport
  Bus Creator20 : BusCreator
  Bus Selector8 : BusSelector  OutputSignals=signal1,signal2,signal3,signal4
  gateway21 : Subsystem
  power{20..23} (4 alike) : casper_library_misc/power  BitWidth=18  add_latency=2  mult_latency=3
  Out1 : Outport
  wires:
  Bus Selector8/2 -> power21/1  "<signal2>"
  Bus Selector8/3 -> power22/1  "<signal3>"
  Bus Creator20/1 -> gateway21/1(data[4])
  power22/1 -> Bus Creator20/3
  power23/1 -> Bus Creator20/4
  In1/1 -> Bus Selector8/1
  power20/1 -> Bus Creator20/1
  power21/1 -> Bus Creator20/2
  Bus Selector8/1 -> power20/1  "<signal1>"
  Bus Selector8/4 -> power23/1  "<signal4>"
  gateway21/1(to_scope) -> Out1/1

== system adc16_dbf_4fft/bus_power2scope1 ==
  In1 : Inport
  Bus Creator20 : BusCreator
  Bus Selector8 : BusSelector  OutputSignals=signal1,signal2,signal3,signal4
  gateway21 : Subsystem
  power{20..23} (4 alike) : casper_library_misc/power  BitWidth=18  add_latency=2  mult_latency=3
  Out1 : Outport
  wires:
  gateway21/1(to_scope) -> Out1/1
  Bus Selector8/4 -> power23/1  "<signal4>"
  Bus Selector8/1 -> power20/1  "<signal1>"
  power21/1 -> Bus Creator20/2
  power20/1 -> Bus Creator20/1
  In1/1 -> Bus Selector8/1
  power23/1 -> Bus Creator20/4
  power22/1 -> Bus Creator20/3
  Bus Creator20/1 -> gateway21/1(data[4])
  Bus Selector8/3 -> power22/1  "<signal3>"
  Bus Selector8/2 -> power21/1  "<signal2>"

== system adc16_dbf_4fft/bus_power2scope2 ==
  In1 : Inport
  Bus Creator20 : BusCreator
  Bus Selector8 : BusSelector  OutputSignals=signal1,signal2,signal3,signal4
  gateway21 : Subsystem
  power{20..23} (4 alike) : casper_library_misc/power  BitWidth=18  add_latency=2  mult_latency=3
  Out1 : Outport
  wires:
  Bus Selector8/2 -> power21/1  "<signal2>"
  Bus Selector8/3 -> power22/1  "<signal3>"
  Bus Creator20/1 -> gateway21/1(data[4])
  power22/1 -> Bus Creator20/3
  power23/1 -> Bus Creator20/4
  In1/1 -> Bus Selector8/1
  power20/1 -> Bus Creator20/1
  power21/1 -> Bus Creator20/2
  Bus Selector8/1 -> power20/1  "<signal1>"
  Bus Selector8/4 -> power23/1  "<signal4>"
  gateway21/1(to_scope) -> Out1/1

== system adc16_dbf_4fft/bus_power2scope3 ==
  In1 : Inport
  Bus Creator20 : BusCreator
  Bus Selector8 : BusSelector  OutputSignals=signal1,signal2,signal3,signal4
  gateway21 : Subsystem
  power{20..23} (4 alike) : casper_library_misc/power  BitWidth=18  add_latency=2  mult_latency=3
  Out1 : Outport
  wires:
  gateway21/1(to_scope) -> Out1/1
  Bus Selector8/4 -> power23/1  "<signal4>"
  Bus Selector8/1 -> power20/1  "<signal1>"
  power21/1 -> Bus Creator20/2
  power20/1 -> Bus Creator20/1
  In1/1 -> Bus Selector8/1
  power23/1 -> Bus Creator20/4
  power22/1 -> Bus Creator20/3
  Bus Creator20/1 -> gateway21/1(data[4])
  Bus Selector8/3 -> power22/1  "<signal3>"
  Bus Selector8/2 -> power21/1  "<signal2>"

== system adc16_dbf_4fft/gateway ==
  data_a : Inport
  data_b : Inport  Port=2
  data_c : Inport  Port=3
  data_d : Inport  Port=4
  Bus Creator : BusCreator  Inputs=16
  Bus Selector : BusSelector  OutputSignals=a1,a2,a3,a4
  Bus Selector1 : BusSelector  OutputSignals=b1,b2,b3,b4
  Bus Selector2 : BusSelector  OutputSignals=c1,c2,c3,c4
  Bus Selector3 : BusSelector  OutputSignals=d1,d2,d3,d4
  Gateway Out{,1..15} (16 alike) : xbsIndex_r4/Gateway Out  inherit_from_input=off  hdl_port=on  timing_constraint=None  locs_specified=off  LOCs={}  UseAsDAC=off  DACChannel='1'  block_type=gatewayout
  to_scope : Outport
  wires:
  data_a/1 -> Bus Selector/1
  Bus Selector3/4 -> Gateway Out13/1  "<d4>"
  Bus Selector3/3 -> Gateway Out12/1  "<d3>"
  Bus Selector3/2 -> Gateway Out15/1  "<d2>"
  Bus Selector3/1 -> Gateway Out14/1  "<d1>"
  Bus Selector2/4 -> Gateway Out11/1  "<c4>"
  Bus Selector2/3 -> Gateway Out10/1  "<c3>"
  Bus Selector2/2 -> Gateway Out9/1  "<c2>"
  Bus Selector2/1 -> Gateway Out8/1  "<c1>"
  Bus Selector1/2 -> Gateway Out5/1  "<b2>"
  Bus Selector1/1 -> Gateway Out4/1  "<b1>"
  Bus Selector1/4 -> Gateway Out7/1  "<b4>"
  Bus Selector1/3 -> Gateway Out6/1  "<b3>"
  Bus Selector/4 -> Gateway Out3/1  "<a4>"
  Bus Selector/2 -> Gateway Out1/1  "<a2>"
  Bus Selector/1 -> Gateway Out/1  "<a1>"
  Bus Selector/3 -> Gateway Out2/1  "<a3>"
  Bus Creator/1 -> to_scope/1
  Gateway Out4/1 -> Bus Creator/5
  Gateway Out11/1 -> Bus Creator/12
  Gateway Out10/1 -> Bus Creator/11
  Gateway Out5/1 -> Bus Creator/6
  Gateway Out9/1 -> Bus Creator/10
  Gateway Out6/1 -> Bus Creator/7
  Gateway Out8/1 -> Bus Creator/9
  Gateway Out13/1 -> Bus Creator/16
  Gateway Out/1 -> Bus Creator/1
  Gateway Out7/1 -> Bus Creator/8
  Gateway Out1/1 -> Bus Creator/2
  Gateway Out12/1 -> Bus Creator/15
  Gateway Out15/1 -> Bus Creator/14
  Gateway Out2/1 -> Bus Creator/3
  Gateway Out3/1 -> Bus Creator/4
  Gateway Out14/1 -> Bus Creator/13
  data_b/1 -> Bus Selector1/1
  data_c/1 -> Bus Selector2/1
  data_d/1 -> Bus Selector3/1

== system adc16_dbf_4fft/gateway1 ==
  data[4] : Inport
  Bus Creator : BusCreator
  Bus Selector : BusSelector  OutputSignals=signal1,signal2,signal3,signal4
  Gateway Out{,1..3} (4 alike) : xbsIndex_r4/Gateway Out  inherit_from_input=off  hdl_port=on  timing_constraint=None  locs_specified=off  LOCs={}  UseAsDAC=off  DACChannel='1'  block_type=gatewayout
  to_scope : Outport
  wires:
  Gateway Out3/1 -> Bus Creator/4
  Gateway Out2/1 -> Bus Creator/3
  Gateway Out1/1 -> Bus Creator/2
  Gateway Out/1 -> Bus Creator/1
  Bus Creator/1 -> to_scope/1
  Bus Selector/3 -> Gateway Out2/1  "<signal3>"
  Bus Selector/1 -> Gateway Out/1  "<signal1>"
  Bus Selector/2 -> Gateway Out1/1  "<signal2>"
  Bus Selector/4 -> Gateway Out3/1  "<signal4>"
  data[4]/1 -> Bus Selector/1
